simulink model "rct_pendulum_LQ_EKF_SwingUp"  (R2025b)
settings: Solver=ode4  StartTime=0.0  StopTime=20  FixedStep=0.01  RelTol=1e-3
values from neighbouring files (symbols this model uses):
  L = [-9.66097161261 -12.9704114691 -67.2769198673 -12.1965045207]    [cartpole_cfg.mat]    (also in cartpole_setup.m = lqr_riccati(F, W, V, P, 1e-12, 10000); lqr_riccati.m = (P + W'*T*W) \ (W'*T*F))
  m = p.m    [cartpole_dynamics.m]    (also in cartpole_setup.m = 0.2; run_mpc_optimization.m = 0.2)
  N = length(u_opt)    [compare_plan_vs_real.m]    (also in fh_controller.m = 100; iLQR_controller.m = 100; run_mpc_optimization.m = 40)
  s = sin(th)    [cartpole_dynamics.m]    (also in run_mpc_optimization.m)
  Ts = 0.01    [cartpole_cfg.mat]    (also in cartpole_setup.m; compare_plan_vs_real.m = Ts_swing; fh_controller.m = Ts_swing; iLQR_controller.m = Ts_swing)
undefined symbols (not defined in the file or in its folder): X, Y, Z
libraries: sm_lib x10, nesl_utility x3, simulink x1
settings Model: Creator=charbel  LastModifiedBy=charbel

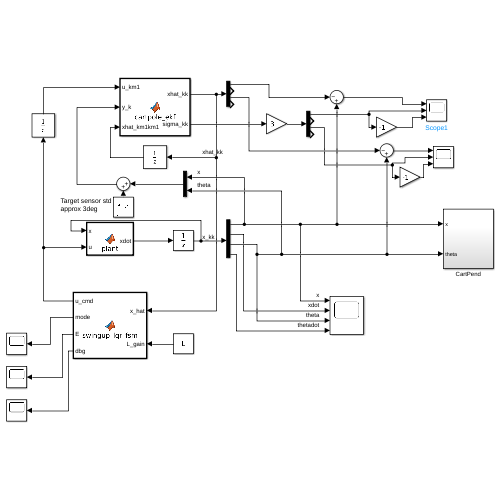
[thumbnail: Simulink's stored preview of the top-level diagram]
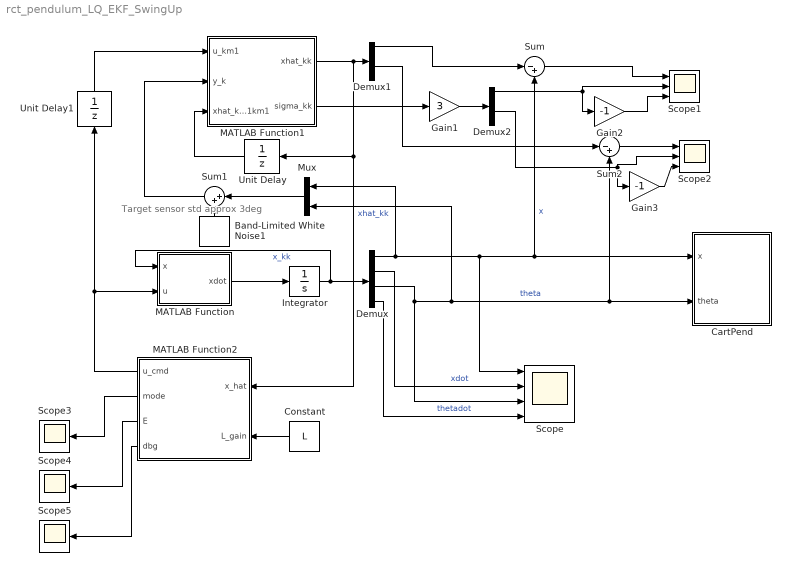
== system rct_pendulum_LQ_EKF_SwingUp ==
  note: Target sensor std approx 3deg
  Band-Limited White Noise1 : simulink/Sources/Band-Limited White Noise  Cov=[2.5e-5, 2.5e-5]  Ts=Ts  seed=[23341]
  CartPend : Subsystem
  Constant : Constant  Value=L
  Demux : Demux
  Demux1 : Demux
  Demux2 : Demux
  Gain1 : Gain  Gain=3
  Gain2 : Gain  Gain=-1
  Gain3 : Gain  Gain=-1
  Integrator : Integrator  InitialCondition=[0;0;pi-0.1;0]
  MATLAB Function : MATLAB Function  TreatAsAtomicUnit=on
  MATLAB Function1 : MATLAB Function  TreatAsAtomicUnit=on
  MATLAB Function2 : MATLAB Function  TreatAsAtomicUnit=on
  Mux : Mux  Inputs=2
  Scope : Scope  NumInputPorts=4
      settings: ActiveDisplayYMinimum=-1.6293023190885179  ActiveDisplayYMaximum=1.5525793691837841
  Scope1 : Scope  NumInputPorts=3
      settings: ActiveDisplayYMinimum=-0.60194595187691524  ActiveDisplayYMaximum=0.33293839527305474
  Scope2 : Scope  NumInputPorts=3
      settings: ActiveDisplayYMinimum=-1.8467574942470184  ActiveDisplayYMaximum=1.1043695196306278  DataLoggingVariableName=ScopeData2
  Scope3 : Scope
      settings: ActiveDisplayYMinimum=-0.63806002049509658  ActiveDisplayYMaximum=1.7190014074089537  DataLoggingVariableName=ScopeData3
  Scope4 : Scope
      settings: ActiveDisplayYMinimum=-0.51472739469992612  ActiveDisplayYMaximum=0.20308421876544905  DataLoggingVariableName=ScopeData4
  Scope5 : Scope
      settings: ActiveDisplayYMinimum=-17.763248275384178  ActiveDisplayYMaximum=15.648939556509045  DataLoggingVariableName=ScopeData5
  Sum : Sum  Inputs=|-+
  Sum1 : Sum  Inputs=|++
  Sum2 : Sum  Inputs=|-+
  Unit Delay : UnitDelay  SampleTime=0.01  HasFrameUpgradeWarning=on
  Unit Delay1 : UnitDelay  SampleTime=0.01  HasFrameUpgradeWarning=on
  wires:
  Unit Delay/1 -> MATLAB Function1/3(xhat_km1km1)
  Unit Delay1/1 -> MATLAB Function1/1(u_km1)
  MATLAB Function1/1(xhat_kk) -> Demux1/1, MATLAB Function2/1(x_hat), Unit Delay/1  "xhat_kk"
  Mux/1 -> Sum1/1
  Sum1/1 -> MATLAB Function1/2(y_k)
  Integrator/1 -> MATLAB Function/1(x), Demux/1  "x_kk"
  Demux/3 -> Scope/3, Mux/2, CartPend/2(theta), Sum2/2  "theta"
  Demux/2 -> Scope/2  "xdot"
  Demux/1 -> Mux/1, Sum/2, CartPend/1(x), Scope/1  "x"
  Demux/4 -> Scope/4  "thetadot"
  MATLAB Function2/1(u_cmd) -> MATLAB Function/2(u), Unit Delay1/1
  Band-Limited White Noise1/1 -> Sum1/2
  MATLAB Function/1(xdot) -> Integrator/1
  Sum/1 -> Scope1/1
  MATLAB Function1/2(sigma_kk) -> Gain1/1
  Demux1/1 -> Sum/1
  Gain1/1 -> Demux2/1
  Demux2/1 -> Gain2/1, Scope1/2
  Gain2/1 -> Scope1/3
  Demux1/3 -> Sum2/1
  Sum2/1 -> Scope2/1
  Demux2/3 -> Gain3/1, Scope2/2
  Gain3/1 -> Scope2/3
  Constant/1 -> MATLAB Function2/2(L_gain)
  MATLAB Function2/2(mode) -> Scope3/1
  MATLAB Function2/3(E) -> Scope4/1
  MATLAB Function2/4(dbg) -> Scope5/1

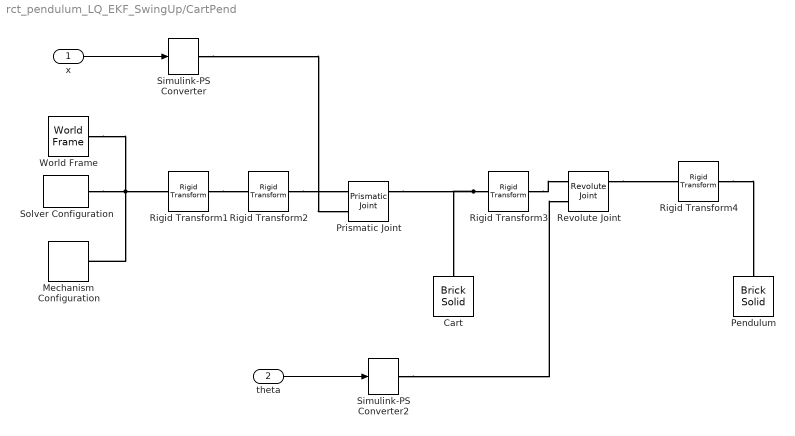
== system rct_pendulum_LQ_EKF_SwingUp/CartPend ==
  x : Inport
  theta : Inport  Port=2
  Cart : sm_lib/Body Elements/Brick Solid  BrickDimensions=[0.3/6, 0.3/6, 0.3/3]  BrickDimensionsUnits=m  ExportEntireGeometry=off  InertiaType=PointMass  BasedOnType=Mass  Density=1000  DensityUnits=kg/(m^3)  Mass=0.5  MassUnits=kg  CenterOfMass=[0 0 0]  CenterOfMassUnits=m  MomentsOfInertia=[1 1 1]  MomentsOfInertiaUnits=kg*m^2  ProductsOfInertia=[0 0 0]  ProductsOfInertiaUnits=kg*m^2  GraphicType=FromGeometry  MarkerShape=Sphere  MarkerSize=10  GraphicVisPropType=SimpleVisualProperties  GraphicDiffuseColor=[0.5 0.5 0.5]  GraphicOpacity=1.0  GraphicSpecularColor=[0.5 0.5 0.5 1.0]  GraphicAmbientColor=[0.15 0.15 0.15 1.0]  GraphicEmissiveColor=[0.0 0.0 0.0 1.0]  GraphicShininess=75  DoExposeReferenceFrame=on  SerializedFrames=<Frames/>
  Mechanism Configuration : sm_lib/Utilities/Mechanism Configuration  UniformGravity=Constant  GravityVector=[0 0 -9.81]  GravityVectorUnits=m/s^2  LinearizationDelta=0.001  JointModeTransitionNonlinearIterations=2
  Pendulum : sm_lib/Body Elements/Brick Solid  BrickDimensions=[0.3, 0.3/12, 0.3/12]  BrickDimensionsUnits=m  ExportEntireGeometry=off  InertiaType=PointMass  BasedOnType=Mass  Density=1000  DensityUnits=kg/(m^3)  Mass=0.2  MassUnits=kg  CenterOfMass=[0 0 0]  CenterOfMassUnits=m  MomentsOfInertia=[1 1 1]  MomentsOfInertiaUnits=kg*m^2  ProductsOfInertia=[0 0 0]  ProductsOfInertiaUnits=kg*m^2  GraphicType=FromGeometry  MarkerShape=Sphere  MarkerSize=10  GraphicVisPropType=SimpleVisualProperties  GraphicDiffuseColor=[0.8 0.0 0.2]  GraphicOpacity=1.0  GraphicSpecularColor=[0.5 0.5 0.5 1.0]  GraphicAmbientColor=[0.15 0.15 0.15 1.0]  GraphicEmissiveColor=[0.0 0.0 0.0 1.0]  GraphicShininess=75  DoExposeReferenceFrame=on  SerializedFrames=<Frames/>
  Prismatic Joint : sm_lib/Joints/Prismatic Joint  JointMode=Normal  CompositeWrenchDir=FollowerOnBase  CompositeWrenchFrame=BaseFrame  SenseConstraintForce=off  SenseConstraintTorque=off  SenseTotalForce=off  SenseTotalTorque=off  PositionTargetSpecify=off  PositionTargetPriority=High  PositionTargetValue=0  PositionTargetValueUnits=m  VelocityTargetSpecify=off  VelocityTargetPriority=High  VelocityTargetValue=0  VelocityTargetValueUnits=m/s  EquilibriumPosition=0  EquilibriumPositionUnits=m  SpringStiffness=0  SpringStiffnessUnits=N/m  DampingCoefficient=0.1  DampingCoefficientUnits=N/(m/s)  LowerLimitSpecify=off  LowerLimitBound=-1  LowerLimitBoundUnits=m  LowerLimitStiffness=1e6  LowerLimitStiffnessUnits=N/m  LowerLimitDamping=1e3  LowerLimitDampingUnits=N/(m/s)  LowerLimitTransitionRegionWidth=1e-4  LowerLimitTransitionRegionWidthUnits=m  UpperLimitSpecify=off  UpperLimitBound=1  UpperLimitBoundUnits=m  UpperLimitStiffness=1e6  UpperLimitStiffnessUnits=N/m  UpperLimitDamping=1e3  UpperLimitDampingUnits=N/(m/s)  UpperLimitTransitionRegionWidth=1e-4  UpperLimitTransitionRegionWidthUnits=m  TorqueActuationMode=ComputedTorque  MotionActuationMode=InputMotion  SensePosition=on  SenseVelocity=off  SenseAcceleration=off  SenseTorqueForce=off  SenseLowerLimitTorqueForce=off  SenseUpperLimitTorqueForce=off
  Revolute Joint : sm_lib/Joints/Revolute Joint  JointMode=Normal  CompositeWrenchDir=FollowerOnBase  CompositeWrenchFrame=BaseFrame  SenseConstraintForce=off  SenseConstraintTorque=off  SenseTotalForce=off  SenseTotalTorque=off  PositionTargetSpecify=off  PositionTargetPriority=High  PositionTargetValue=theta0  PositionTargetValueUnits=deg  VelocityTargetSpecify=off  VelocityTargetPriority=High  VelocityTargetValue=0  VelocityTargetValueUnits=deg/s  EquilibriumPosition=0  EquilibriumPositionUnits=deg  SpringStiffness=0  SpringStiffnessUnits=N*m/deg  DampingCoefficient=0  DampingCoefficientUnits=N*m/(rad/s)  LowerLimitSpecify=off  LowerLimitBound=-90  LowerLimitBoundUnits=deg  LowerLimitStiffness=1e4  LowerLimitStiffnessUnits=N*m/deg  LowerLimitDamping=10  LowerLimitDampingUnits=N*m/(deg/s)  LowerLimitTransitionRegionWidth=0.1  LowerLimitTransitionRegionWidthUnits=deg  UpperLimitSpecify=off  UpperLimitBound=90  UpperLimitBoundUnits=deg  UpperLimitStiffness=1e4  UpperLimitStiffnessUnits=N*m/deg  UpperLimitDamping=10  UpperLimitDampingUnits=N*m/(deg/s)  UpperLimitTransitionRegionWidth=0.1  UpperLimitTransitionRegionWidthUnits=deg  TorqueActuationMode=ComputedTorque  MotionActuationMode=InputMotion  SensePosition=on  SenseVelocity=off  SenseAcceleration=off  SenseTorqueForce=off  SenseLowerLimitTorqueForce=off  SenseUpperLimitTorqueForce=off
  Rigid Transform1 : sm_lib/Frames and Transforms/Rigid Transform  RotationMethod=StandardAxis  FollAlignAxisA=+X  BaseAlignAxisA=+Y  FollAlignAxisB=+Y  BaseAlignAxisB=+Z  RotationStandardAxis=+Y  RotationAngle=90  RotationAngleUnits=deg  RotationArbitraryAxis=[0 0 1]  RotationSequenceAxes=FollowerAxes  RotationSequence=XYX  RotationSequenceAngles=[0 0 0]  RotationSequenceAnglesUnits=deg  RotationMatrix=[1 0 0; 0 1 0; 0 0 1]  Quaternion=[1 0 0 0]  TranslationMethod=None  TranslationCartesianOffset=[0 0 0]  TranslationCartesianOffsetUnits=m  TranslationStandardAxis=+Z  TranslationStandardOffset=0  TranslationStandardOffsetUnits=m  TranslationROffset=0  TranslationROffsetUnits=m  TranslationThetaOffset=0  TranslationThetaOffsetUnits=deg  TranslationZOffset=0  TranslationZOffsetUnits=m
  Rigid Transform2 : sm_lib/Frames and Transforms/Rigid Transform  RotationMethod=StandardAxis  FollAlignAxisA=+X  BaseAlignAxisA=+Y  FollAlignAxisB=+Y  BaseAlignAxisB=+Z  RotationStandardAxis=+Z  RotationAngle=180  RotationAngleUnits=deg  RotationArbitraryAxis=[0 0 1]  RotationSequenceAxes=FollowerAxes  RotationSequence=XYX  RotationSequenceAngles=[0 0 0]  RotationSequenceAnglesUnits=deg  RotationMatrix=[1 0 0; 0 1 0; 0 0 1]  Quaternion=[1 0 0 0]  TranslationMethod=None  TranslationCartesianOffset=[0 0 0]  TranslationCartesianOffsetUnits=m  TranslationStandardAxis=+Z  TranslationStandardOffset=0  TranslationStandardOffsetUnits=m  TranslationROffset=0  TranslationROffsetUnits=m  TranslationThetaOffset=0  TranslationThetaOffsetUnits=deg  TranslationZOffset=0  TranslationZOffsetUnits=m
  Rigid Transform3 : sm_lib/Frames and Transforms/Rigid Transform  RotationMethod=StandardAxis  FollAlignAxisA=+X  BaseAlignAxisA=+Y  FollAlignAxisB=+Y  BaseAlignAxisB=+Z  RotationStandardAxis=-X  RotationAngle=90  RotationAngleUnits=deg  RotationArbitraryAxis=[0 0 1]  RotationSequenceAxes=FollowerAxes  RotationSequence=XYX  RotationSequenceAngles=[0 0 0]  RotationSequenceAnglesUnits=deg  RotationMatrix=[1 0 0; 0 1 0; 0 0 1]  Quaternion=[1 0 0 0]  TranslationMethod=None  TranslationCartesianOffset=[0 0 0]  TranslationCartesianOffsetUnits=m  TranslationStandardAxis=+Z  TranslationStandardOffset=0  TranslationStandardOffsetUnits=m  TranslationROffset=0  TranslationROffsetUnits=m  TranslationThetaOffset=0  TranslationThetaOffsetUnits=deg  TranslationZOffset=0  TranslationZOffsetUnits=m
  Rigid Transform4 : sm_lib/Frames and Transforms/Rigid Transform  RotationMethod=StandardAxis  FollAlignAxisA=+X  BaseAlignAxisA=+Y  FollAlignAxisB=+Y  BaseAlignAxisB=+Z  RotationStandardAxis=+X  RotationAngle=90  RotationAngleUnits=deg  RotationArbitraryAxis=[0 0 1]  RotationSequenceAxes=FollowerAxes  RotationSequence=XYX  RotationSequenceAngles=[0 0 0]  RotationSequenceAnglesUnits=deg  RotationMatrix=[1 0 0; 0 1 0; 0 0 1]  Quaternion=[1 0 0 0]  TranslationMethod=StandardAxis  TranslationCartesianOffset=[0 0 0]  TranslationCartesianOffsetUnits=m  TranslationStandardAxis=+X  TranslationStandardOffset=0.3/2  TranslationStandardOffsetUnits=m  TranslationROffset=0  TranslationROffsetUnits=m  TranslationThetaOffset=0  TranslationThetaOffsetUnits=deg  TranslationZOffset=0  TranslationZOffsetUnits=m
  Simulink-PS Converter : nesl_utility/Simulink-PS Converter  PhysicalDomain=network_engine_domain  SubClassName=ps_input  LeftPortType=input  RightPortType=output  PseudoPeriodic=off  Frequencies=[]  NoiseDistribution=none  NoiseParameters=[]  Unit=1  AffineConversion=off  FilteringAndDerivatives=zero  SimscapeFilterOrder=1  InputFilterTimeConstant=0.001  UdotUserProvided=1
  Simulink-PS Converter2 : nesl_utility/Simulink-PS Converter  PhysicalDomain=network_engine_domain  SubClassName=ps_input  LeftPortType=input  RightPortType=output  PseudoPeriodic=off  Frequencies=[]  NoiseDistribution=none  NoiseParameters=[]  Unit=1  AffineConversion=off  FilteringAndDerivatives=zero  SimscapeFilterOrder=1  InputFilterTimeConstant=0.001  UdotUserProvided=1
  Solver Configuration : nesl_utility/Solver Configuration  PhysicalDomain=network_engine_domain  SubClassName=solver  LeftPortType=input  RightPortType=generic  Tones=[]  Harmonics=[]  SimulateNoise=off  Profile=off  UseLocalSampling=off  EnableSwitchedLinearOptims=on  FrequencyDomain=off  UseCCode=off  RelTol=0.001  AbsTol=1e-06  MinStep=1e-09  ToWorkspace=off  RevertToSquareIcSolve=off  NumHomotopyIterations=100  PhasorMode=off  PhasorModeNumHarmonics=1  ConsistencySolver=NEWTON_FTOL  IndexReductionMethod=DerivativeReplacement  DoDC=off  ResidualTolerance=1e-09  ConsistencyTolSource=GLOBAL  ConsistencyAbsTol=0.001  ConsistencyRelTol=0.001  ConsistencyTolFactor=0.001  UseLocalSolver=off  LocalSolverChoice=NE_BACKWARD_EULER_ADVANCER  ResolveIndetEquations=on  FunctionEvalNumThread=1  LocalSolverSampleTime=0.001  DoFixedCost=off  MaxNonlinIter=3  MaxModeIter=2  ComputeImpulses=off  ImpulseIterations=2  LinearAlgebra=Sparse  LinearAlgebraNumThread=0  EquationFormulation=NE_TIME_EF  DelaysMemoryBudget=1024  AutomaticFiltering=on  FilteringTimeConstant=0.001  PartitionStorageMethod=AS_NEEDED  PartitionMemoryBudget=1024  PartitionMethod=FAST  MultibodyUseLocalSolver=off  MultibodyLocalSolverChoice=ODE1  MultibodyLocalSolverSampleTime=0.001
  World Frame : sm_lib/Frames and Transforms/World Frame
  wires:
  x/1 -> Simulink-PS Converter/1
  theta/1 -> Simulink-PS Converter2/1
  connections:
  Rigid Transform3/LConn1 -- Cart/RConn1 -- Prismatic Joint/RConn1
  World Frame/RConn1 -- Solver Configuration/RConn1 -- Mechanism Configuration/RConn1 -- Rigid Transform1/LConn1
  Revolute Joint/RConn1 -- Rigid Transform4/LConn1
  Rigid Transform4/RConn1 -- Pendulum/RConn1
  Rigid Transform3/RConn1 -- Revolute Joint/LConn1
  Rigid Transform1/RConn1 -- Rigid Transform2/LConn1
  Rigid Transform2/RConn1 -- Prismatic Joint/LConn1
  Simulink-PS Converter2/RConn1 -- Revolute Joint/LConn2
  Simulink-PS Converter/RConn1 -- Prismatic Joint/LConn2

== matlab function rct_pendulum_LQ_EKF_SwingUp/MATLAB Function1 ==
  settings: updateMethod=DISCRETE  sampleTime=0.01
  data: u_km1 input size=1; xhat_kk output double size=4; y_k input double size=2; xhat_km1km1 input double size=4; sigma_kk output
function [xhat_kk, sigma_kk] = cartpole_ekf(u_km1, y_k, xhat_km1km1) 
    assert(all(size(xhat_km1km1) == [4 1]));
    assert(all(size(y_k)         == [2 1]));
    assert(all(size(u_km1)       == [1 1]));

    p.M = 0.5; p.m = 0.2; p.l = 0.3; p.b = 0.1; p.g = 9.81;
    Ts  = 0.01;

    G = [1 0 0 0;
         0 0 1 0];

    Q  = diag([1e-5 1e-4 1e-5 1e-4]);
    R  = diag([2.5e-3 2.5e-3]); % R ≈ diag([σ_pos², σ_theta²]) = diag([NoisePower_pos/Ts, NoisePower_theta/Ts])
    P0 = diag([5 5 5 5]);
    n  = 4;
    ep = 1e-6; 

    persistent Sigma
    if isempty(Sigma)
        Sigma = P0;
    end

    % Prediction & Rk4 discretization
    k1 = cartpole_dynamics(xhat_km1km1, u_km1, p);
    k2 = cartpole_dynamics(xhat_km1km1 + (Ts/2)*k1, u_km1, p);
    k3 = cartpole_dynamics(xhat_km1km1 + (Ts/2)*k2, u_km1, p);
    k4 = cartpole_dynamics(xhat_km1km1 + Ts*k3, u_km1, p);
    xhat_kkm1 = xhat_km1km1 + (Ts/6)*(k1 + 2*k2 + 2*k3 + k4);


    F = zeros(n,n);
    for i = 1:n
        e  = zeros(n,1); e(i) = ep;
        fp = (xhat_km1km1+e) + Ts*cartpole_dynamics(xhat_km1km1+e, u_km1, p);
        fm = (xhat_km1km1-e) + Ts*cartpole_dynamics(xhat_km1km1-e, u_km1, p);
        F(:,i) = (fp - fm)/(2*ep);
    end
    Sigma_kkm1 = F*Sigma*F.' + Q;

    % Estimation
    yhat_kkm1 = G*xhat_kkm1;
    S  = G*Sigma_kkm1*G.' + R;
    Hk = (Sigma_kkm1*G.')/S;

    xhat_kk = zeros(4,1);
    xhat_kk(:) = xhat_kkm1 + Hk*(y_k - yhat_kkm1);

    Sigma = Sigma_kkm1 - Hk*S*Hk.';
    Sigma = 0.5*(Sigma + Sigma.');

    sigma_kk = zeros(4,1);                  
    sigma_kk(:) = sqrt(diag(Sigma));        
end

function xdot = cartpole_dynamics(x, u, p)
    vel = x(2); th = x(3); om = x(4);
    M = p.M; m = p.m; l = p.l; b = p.b; g = p.g;
    F = u(1);
    s = sin(th); c = cos(th);
    den    = M + m*s^2;
    common = F - b*vel + m*l*s*om^2;
    xacc   = ( common - m*g*c*s ) / den;
    thacc  = ( (M+m)*g*s - c*common ) / (l*den);
    xdot   = [ vel ; xacc ; om ; thacc ];
end

== matlab function rct_pendulum_LQ_EKF_SwingUp/MATLAB Function ==
  data: x input; u input; xdot output
function xdot = plant(x,u)
    p.M = 0.5; p.m = 0.2; p.l = 0.3; p.b = 0.1; p.g = 9.81;
    xdot = zeros(4,1);               
    xdot(:) = cartpole_dynamics(x,u,p);
end

== matlab function rct_pendulum_LQ_EKF_SwingUp/MATLAB Function2 ==
  settings: updateMethod=DISCRETE  sampleTime=0.01
  data: x_hat input double size=4; u_cmd output; L_gain input double size=4; mode output; E output; dbg output
function [u_cmd, mode, E, dbg] = swingup_lqr_fsm(x_hat, L_gain)
%SWINGUP_LQR_FSM  Energy swing-up -> LQR catch, with diagnostics.
%   Outputs: u_cmd, mode(0/1), E(energy), dbg=[theta_w; omega; cart_pos]
%   Scope E and dbg, zoom into a mode=1 pulse, and read off WHY it drops.

    assert(all(size(x_hat) == [4 1]));
    assert(numel(L_gain) == 4);
    L_gain = reshape(L_gain, 1, 4);

    % ============================ TUNING ============================
    m = 0.2;  l = 0.3;  g = 9.81;

    k_E  = 15.0;     % PUMP. Too low: never reaches top. Too high (16!):
                    %       over-rotates, cart runs away, catch fails.
                    %       Sweep DOWN from 16 to find a gentle arrival.
    kp_x = 4.0;     % centering: raise if the cart runs away during swing
    kd_x = 4.0;

    F_MAX = 15.0;

    CATCH_ANGLE = 0.50;   % enter BALANCE below this angle  (~11 deg)
    CATCH_VEL   = 1.4;    % ...and only if SLOW. Lower = cleaner catch,
                          %    but needs a gentle k_E so the apex is slow.
    FALL_ANGLE  = 0.50;   % leave BALANCE above this angle
    % ===============================================================

    pos = x_hat(1);  vel = x_hat(2);  theta = x_hat(3);  omega = x_hat(4);
    theta_w = atan2(sin(theta), cos(theta));

    persistent state
    if isempty(state), state = 0; end
    if state == 0
        if (abs(theta_w) < CATCH_ANGLE) && (abs(omega) < CATCH_VEL)
            state = 1;
        end
    else
        if abs(theta_w) > FALL_ANGLE
            state = 0;
        end
    end
    mode = state;

    % energy (always computed, for logging)
    E = 0.5*m*(l*omega)^2 + m*g*l*(cos(theta_w) - 1);   % target 0 at top

    if state == 1
        u = -L_gain * x_hat;
    else
        u_swing  = k_E * E * omega * cos(theta_w);
        u_center = -kp_x * pos - kd_x * vel;
        u = u_swing + u_center;
    end

    u_cmd = max(min(u, F_MAX), -F_MAX);
    dbg = [theta_w; omega; pos];
end
